simulink model "ProyectoGlobal_AyCD_Cantu_LagoTejo"  (R2021a)
settings: Solver=ode23  StartTime=0.0  StopTime=inf  MinStep=1e-4
values from neighbouring files (symbols this model uses):
  a_hMax = 0.75    [Datos_ProyectoGlobal_AyCD_Cantu_LagoTejo.m]    (also in Datos_v18.m; PID_calculado.mat)
  a_tMax = 0.8    [Datos_ProyectoGlobal_AyCD_Cantu_LagoTejo.m]    (also in Datos_v18.m; PID_calculado.mat)
  b_cx = 1e6    (= 1000000)    [Datos_ProyectoGlobal_AyCD_Cantu_LagoTejo.m]    (also in Datos_v18.m; PID_calculado.mat)
  b_cy = 1e7    (= 10000000)    [Datos_ProyectoGlobal_AyCD_Cantu_LagoTejo.m]    (also in Datos_v18.m; PID_calculado.mat)
  b_eq_h = ((b_hd + b_hm*(i_h^2))*2/(r_hd^2))    (= 31004.4444444)    [Datos_ProyectoGlobal_AyCD_Cantu_LagoTejo.m]    (also in Datos_v18.m; PID_calculado.mat)
  b_eq_t = ((b_td + b_tm*(i_t^2))/(r_td^2))    (= 21607.2)    [Datos_ProyectoGlobal_AyCD_Cantu_LagoTejo.m]    (also in Datos_v18.m; PID_calculado.mat)
  b_hb = 1e8    (= 100000000)    [Datos_ProyectoGlobal_AyCD_Cantu_LagoTejo.m]    (also in Datos_v18.m; PID_calculado.mat)
  b_hEb = 2.2e9    (= 2200000000)    [Datos_ProyectoGlobal_AyCD_Cantu_LagoTejo.m]    (also in Datos_v18.m; PID_calculado.mat)
  b_t = 90    [Datos_ProyectoGlobal_AyCD_Cantu_LagoTejo.m]    (also in Datos_v18.m; PID_calculado.mat)
  b_tb = 5e6    (= 5000000)    [Datos_ProyectoGlobal_AyCD_Cantu_LagoTejo.m]    (also in Datos_v18.m; PID_calculado.mat)
  b_tw = 3e3    (= 3000)    [Datos_ProyectoGlobal_AyCD_Cantu_LagoTejo.m]    (also in Datos_v18.m; PID_calculado.mat)
  b_wu = 150    [Datos_ProyectoGlobal_AyCD_Cantu_LagoTejo.m]    (also in Datos_v18.m; PID_calculado.mat)
  bah = M_eq_h*n_h*omega_h    [PID_Izaje_B.m]    (also in PID_calculado.mat = 387555.555556)
  bat = M_eq_t*n_t*omega_t    [PID_Carro_B.m]    (also in PID_calculado.mat = 270090)
  CI_h = 5    [Datos_ProyectoGlobal_AyCD_Cantu_LagoTejo.m]    (also in Datos_v18.m; PID_calculado.mat)
  CI_t = -16.25    [Datos_ProyectoGlobal_AyCD_Cantu_LagoTejo.m]    (also in Datos_v18.m; PID_calculado.mat)
  d_t = 1e-3    (= 0.001)    [Datos_ProyectoGlobal_AyCD_Cantu_LagoTejo.m]    (also in Datos_v18.m; PID_calculado.mat)
  g = 9.80665    [Datos_ProyectoGlobal_AyCD_Cantu_LagoTejo.m]    (also in Datos_v18.m; PID_calculado.mat)
  H_c = 2.5    [Datos_ProyectoGlobal_AyCD_Cantu_LagoTejo.m]    (also in Datos_v18.m; PID_calculado.mat)
  i_h = 22    [Datos_ProyectoGlobal_AyCD_Cantu_LagoTejo.m]    (also in Datos_v18.m; PID_calculado.mat)
  i_t = 30    [Datos_ProyectoGlobal_AyCD_Cantu_LagoTejo.m]    (also in Datos_v18.m; PID_calculado.mat)
  k_cy = 1.8e9    (= 1800000000)    [Datos_ProyectoGlobal_AyCD_Cantu_LagoTejo.m]    (also in Datos_v18.m; PID_calculado.mat)
  k_tw = 4.8e5    (= 480000)    [Datos_ProyectoGlobal_AyCD_Cantu_LagoTejo.m]    (also in Datos_v18.m; PID_calculado.mat)
  k_wu = 2.36e8    (= 236000000)    [Datos_ProyectoGlobal_AyCD_Cantu_LagoTejo.m]    (also in Datos_v18.m; PID_calculado.mat)
  Kd_bal = [-2.22044604925e-16 2.22044604925e-16 2.22044604925e-16 0 0 0 0 0 -2.22044604925e-16 0 2.22044604925e-16 -2.22044604925e-16 ... (296091 elements, 501x591)]    [Kp_Kd_balanceo.mat]    (also in PD_Balanceo.m = zeros(length(ML),length(L)))
  Kp_bal = [5.11381136401 5.1081388039 5.10248507909 5.09685008556 5.09123372013 5.08563588037 5.08005646467 5.07449537218 5.06895250283 5.06342775732 5.05792103709 5.05243224433 ... (296091 elements, 501x591)]    [Kp_Kd_balanceo.mat]    (also in PD_Balanceo.m = Kd_bal)
  ksah = M_eq_h*n_h*(omega_h^2)    [PID_Izaje_B.m]    (also in PID_calculado.mat = 922348.374575)
  ksat = M_eq_t*n_t*(omega_t^2)    [PID_Carro_B.m]    (also in PID_calculado.mat = 972648.108)
  ksiah = M_eq_h*n_h*(omega_h^3)    [PID_Izaje_B.m]    (also in PID_calculado.mat = 2195108.57705)
  ksiat = M_eq_t*n_t*(omega_t^3)    [PID_Carro_B.m]    (also in PID_calculado.mat = 3502700.36653)
  lim_xDer = 50    [Datos_ProyectoGlobal_AyCD_Cantu_LagoTejo.m]    (also in Datos_v18.m; PID_calculado.mat)
  lim_xDer_ult = 51    [Datos_ProyectoGlobal_AyCD_Cantu_LagoTejo.m]    (also in Datos_v18.m; PID_calculado.mat)
  lim_xIzq = -30    [Datos_ProyectoGlobal_AyCD_Cantu_LagoTejo.m]    (also in Datos_v18.m; PID_calculado.mat)
  lim_xIzq_ult = -31    [Datos_ProyectoGlobal_AyCD_Cantu_LagoTejo.m]    (also in Datos_v18.m; PID_calculado.mat)
  lim_yInf = -20    [Datos_ProyectoGlobal_AyCD_Cantu_LagoTejo.m]    (also in Datos_v18.m; PID_calculado.mat)
  lim_yInf_ult = -21    [Datos_ProyectoGlobal_AyCD_Cantu_LagoTejo.m]    (also in Datos_v18.m; PID_calculado.mat)
  lim_ySup = 40    [Datos_ProyectoGlobal_AyCD_Cantu_LagoTejo.m]    (also in Datos_v18.m; PID_calculado.mat)
  lim_ySup_ult = 41    [Datos_ProyectoGlobal_AyCD_Cantu_LagoTejo.m]    (also in Datos_v18.m; PID_calculado.mat)
  M_cMax = 50000    [Datos_ProyectoGlobal_AyCD_Cantu_LagoTejo.m]    (also in Datos_v18.m; PID_calculado.mat)
  M_cMin = 2000    [Datos_ProyectoGlobal_AyCD_Cantu_LagoTejo.m]    (also in Datos_v18.m; PID_calculado.mat)
  M_eq_h = (J_hd_hEb+J_hm_hb*i_h^2)*2/r_hd^2    (= 65137.7777778)    [Datos_ProyectoGlobal_AyCD_Cantu_LagoTejo.m]    (also in Datos_v18.m; PID_calculado.mat)
  M_l_max = 32500    [Datos_ProyectoGlobal_AyCD_Cantu_LagoTejo.m]    (also in Datos_v18.m; PID_calculado.mat)
  M_l_nom = 65000    [Datos_ProyectoGlobal_AyCD_Cantu_LagoTejo.m]    (also in Datos_v18.m; PID_calculado.mat)
  M_s = 15000    [Datos_ProyectoGlobal_AyCD_Cantu_LagoTejo.m]    (also in Datos_v18.m; PID_calculado.mat)
  M_t = 30000    [Datos_ProyectoGlobal_AyCD_Cantu_LagoTejo.m]    (also in Datos_v18.m; PID_calculado.mat)
  P_h_nom = 956.15e3    (= 956150)    [Datos_ProyectoGlobal_AyCD_Cantu_LagoTejo.m]    (also in Datos_v18.m; PID_calculado.mat)
  r_hd = 0.75    [Datos_ProyectoGlobal_AyCD_Cantu_LagoTejo.m]    (also in Datos_v18.m; PID_calculado.mat)
  r_td = 0.5    [Datos_ProyectoGlobal_AyCD_Cantu_LagoTejo.m]    (also in Datos_v18.m; PID_calculado.mat)
  T_hbMax = 5e4    (= 50000)    [Datos_ProyectoGlobal_AyCD_Cantu_LagoTejo.m]    (also in Datos_v18.m; PID_calculado.mat)
  T_hEbMax = 1.1e6    (= 1100000)    [Datos_ProyectoGlobal_AyCD_Cantu_LagoTejo.m]    (also in Datos_v18.m; PID_calculado.mat)
  T_hmMax = 2e4    (= 20000)    [Datos_ProyectoGlobal_AyCD_Cantu_LagoTejo.m]    (also in Datos_v18.m; PID_calculado.mat)
  T_tbMax = 5e3    (= 5000)    [Datos_ProyectoGlobal_AyCD_Cantu_LagoTejo.m]    (also in Datos_v18.m; PID_calculado.mat)
  T_tmMax = 3e3    (= 3000)    [Datos_ProyectoGlobal_AyCD_Cantu_LagoTejo.m]    (also in Datos_v18.m; PID_calculado.mat)
  tau_hm = 1e-3    (= 0.001)    [Datos_ProyectoGlobal_AyCD_Cantu_LagoTejo.m]    (also in Datos_v18.m; PID_calculado.mat)
  tau_tm = 1e-3    (= 0.001)    [Datos_ProyectoGlobal_AyCD_Cantu_LagoTejo.m]    (also in Datos_v18.m; PID_calculado.mat)
  v_hMax_0 = 3    [Datos_ProyectoGlobal_AyCD_Cantu_LagoTejo.m]    (also in Datos_v18.m; PID_calculado.mat)
  v_hMax_l = 1.5    [Datos_ProyectoGlobal_AyCD_Cantu_LagoTejo.m]    (also in Datos_v18.m; PID_calculado.mat)
  v_tMax = 4    [Datos_ProyectoGlobal_AyCD_Cantu_LagoTejo.m]    (also in Datos_v18.m; PID_calculado.mat)
  xc = [-28.75 -26.25 -23.75 -21.25 -18.75 -16.25 -13.75 -11.25 -8.75 -6.25 -3.75 -1.25 ... (32 elements, 1x32)]    [PID_calculado.mat]    (also in Perfil_Carga.m = -30+1.25:2.5:50-1.25)
  Y_sb = 15    [Datos_ProyectoGlobal_AyCD_Cantu_LagoTejo.m]    (also in Datos_v18.m; PID_calculado.mat)
  Y_t0 = 45    [Datos_ProyectoGlobal_AyCD_Cantu_LagoTejo.m]    (also in Datos_v18.m; PID_calculado.mat)
  yc = [0 0 0 2.5 0 2.5 0 2.5 0 0 0 0 ... (32 elements, 1x32)]    [PID_calculado.mat]    (also in Perfil_Carga.m = yc2)
undefined symbols (not defined in the file or in its folder): b_eq_td, M_eq_td
libraries: simulink x13
(part 1 of 2)
settings Model: SimulationMode=accelerator  PacingRate=5  Creator=Maxi  LastModifiedBy=maxim
settings SolverCC: InitialStep=1e-3  MaxConsecutiveZCs=10000  MaxConsecutiveMinStep=10000000  ZeroCrossAlgorithm=Adaptive  AlgebraicLoopSolver=TrustRegion
settings DebuggingCC: AlgebraicLoopMsg=none  MaskedZcDiagnostic=none  IgnoredZcDiagnostic=none  SFUnusedDataAndEventsDiag=none  UnderSpecifiedDimensionMsg=warning
settings RTWCC: DLArmComputeVersion=20.02.1

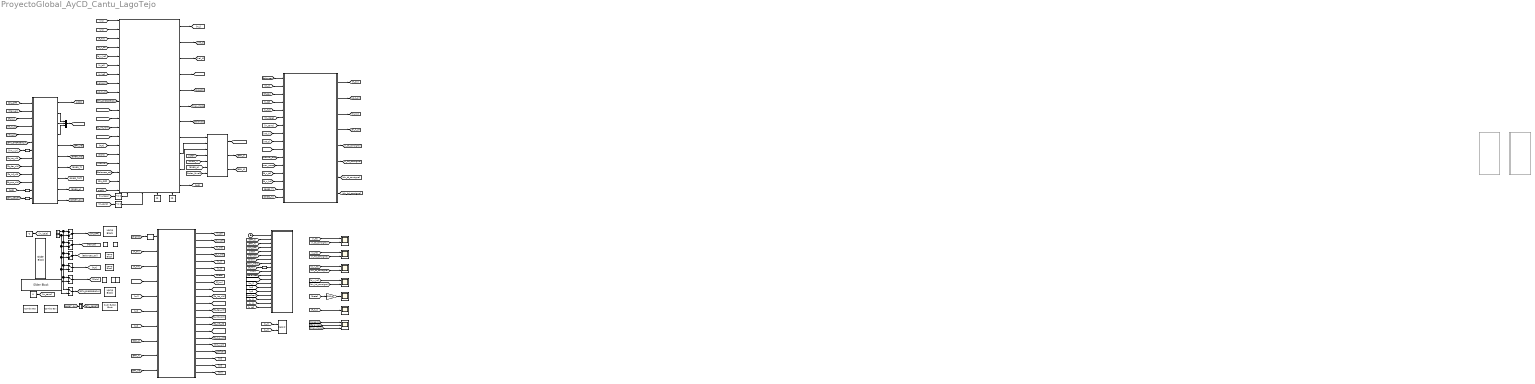
== system ProyectoGlobal_AyCD_Cantu_LagoTejo ==
  note: VISUALIZACION
  note: NIVEL 2
  note: SISTEMA FÍSICO
  note: NIVEL 1
  note: NIVEL 0
  note: HMI
  "  Do" : LampBlock  LabelPosition=Hide
  Angulo de balanceo : Scope
  Automático : LampBlock  LabelPosition=Hide
  Balanceo : LampBlock  LabelPosition=Hide
  Carril Fin : ComboBox  LabelPosition=Hide  SelectedLabel=16
      settings: Values={{'1', '2', '3', '4', '5', '6', '7', '8', '9', '10', '11', '12', '13', '14', '15', '16', '17', '18'}, [1 2 3 4 5 6 7 8 9 10 11 12 13 14 15 16 17 18]}
  Carril Fin Doble : ComboBox  LabelPosition=Hide  SelectedLabel=16
      settings: Values={{'1', '2', '3', '4', '5', '6', '7', '8', '9', '10', '11', '12', '13', '14', '15', '16', '17', '18'}, [1 2 3 4 5 6 7 8 9 10 11 12 13 14 15 16 17 18]}
  Clock2 : Clock
  Compare To Zero : simulink/Logic and Bit Operations/Compare To Zero  relop=>  OutDataTypeStr=boolean
  Compare To Zero2 : simulink/Logic and Bit Operations/Compare To Zero  relop=~=  OutDataTypeStr=boolean
  Compare To Zero7 : simulink/Logic and Bit Operations/Compare To Zero  relop=~=  OutDataTypeStr=boolean
  Constant17 : Constant  Value=0
  Constant18 : Constant
  EMERGENCIA : LampBlock  LabelPosition=Hide
  ENCENDIDO : LampBlock  LabelPosition=Hide
  Estado Final de Frenos : Subsystem
  Estado Final de Frenos10 : Subsystem  Commented=on
  Estado Final de Frenos2 : Subsystem  Commented=on
  Fuerza cable de izaje : Scope
  Gain3 : Gain  Gain=180/pi
  Izaje de carga : Scope  NumInputPorts=2
  MATLAB Function1 : MATLAB Function  TreatAsAtomicUnit=on
  Manual : LampBlock  LabelPosition=Hide
  Manual Switch1 : ManualSwitch  CurrentSetting=0
  Manual Switch2 : ManualSwitch  CurrentSetting=0
  Manual Switch3 : ManualSwitch
  Manual Switch4 : ManualSwitch  CurrentSetting=0
  Manual Switch5 : ManualSwitch
  Manual Switch7 : ManualSwitch
  Memory{5,10,12..13} (4 alike) : Memory
  Modelo Fisico Carro-Izaje-Carga : Subsystem
  Mux7 : Mux  Inputs=3
  Nivel 0 : Stateflow chart  TreatAsAtomicUnit=on
      settings: PortSchema="{\"entries\":[{\"content\":{\"sides\":[{\"content\":{\"connectorIds\":[\"In6\",\"In7\",\"In5\",\"In2\",\"In1\",\"In3\",\"In4\",\"In8\",\"In9\",\"In10\",\"In11\",\"In12\",\"In13\"]},\"type\":\"ConnectorPlacement.EquallySpacedRectSide\",\"uuid\":\"e3679c49-321c-4245-9f4d-6b72d70eef8d\"},{\"content\":{\"connectorIds\":[\"Out1\",\"Out3\",\"Out5\",\"Out4\",\"Out2\",\"Out6\",\"Out7\",\"Out8\",\"Out9\",\"Out10\"],\"side\":\"RIGHT\"},\"type\":\"ConnectorPlacement.EquallySpacedRectSide\",\"uuid\":\"16418e5e-e28d-455d-933a-43b8d78ab460\"},{\"content\":{\"connectorIds\":[],\"side\":\"TOP\"},\"type\":\"ConnectorPlacement.EquallySpacedRectSide\",\"uuid\":\"c85d7e80-ad5f-4217-ba10-6288ee566bb8\"}]},\"type\":\"ConnectorPlacement.EquallySpacedConnector\",\"uuid\":\"c38c6e76-5322-4b57-8473-560e5b1141d3\"}],\"packageUris\":[\"http://schema.mathworks.com/mf0/Connector/R2020b\"],\"version\":\"1.0\"}"
  Nivel 1 : Stateflow chart  TreatAsAtomicUnit=on
      settings: PortSchema="{\"entries\":[{\"content\":{\"sides\":[{\"content\":{\"connectorIds\":[\"In22\",\"In21\",\"In11\",\"In20\",\"In19\",\"In9\",\"In10\",\"In8\",\"In4\",\"In13\",\"In15\",\"In16\",\"In17\",\"In18\",\"In3\",\"In14\",\"In12\",\"In5\",\"In6\",\"In7\"]},\"type\":\"ConnectorPlacement.EquallySpacedRectSide\",\"uuid\":\"68c99711-1ca5-49d6-a421-ad202abad7a3\"},{\"content\":{\"connectorIds\":[\"Out5\",\"Out8\",\"Out6\",\"Out7\",\"Out9\",\"Out11\",\"Out2\",\"Out3\",\"Out4\",\"Out1\",\"Out10\"],\"side\":\"RIGHT\"},\"type\":\"ConnectorPlacement.EquallySpacedRectSide\",\"uuid\":\"bc0f262a-18b8-4d7b-9b7f-403e0cd3788b\"},{\"content\":{\"connectorIds\":[],\"side\":\"TOP\"},\"type\":\"ConnectorPlacement.EquallySpacedRectSide\",\"uuid\":\"2d69c358-e680-43cc-a1d0-9fcf2b39de17\"},{\"content\":{\"connectorIds\":[\"In1\",\"In2\",\"In23\",\"In24\"],\"side\":\"BOTTOM\"},\"type\":\"ConnectorPlacement.EquallySpacedRectSide\",\"uuid\":\"d4a5b5d0-6661-40f6-8d98-5cae5bd8c928\"}]},\"type\":\"ConnectorPlacement.EquallySpacedConnector\",\"uuid\":\"d3c5d26b-109c-4d02-96fa-92f2f1f71ce2\"}],\"packageUris\":[\"http://schema.mathworks.com/mf0/Connector/R2020b\"],\"version\":\"1.0\"}"
  Nivel 2 : Subsystem
  Push Button1 : PushButtonBlock  ButtonText=RESET
  Record : Record  FileSettingsInternal="{\"entries\":[{\"content\":{\"excelSettings\":{\"content\":{},\"type\":\"Streamout.ExcelSettings\"}},\"type\":\"Streamout.FileSettingStorage\",\"uuid\":\"bed3a6e0-7c45-46bb-b7f7-e86d5775e973\"}],\"packageUris\":[\"http://schema.mathworks.com/mf0/streamout_blocks/R2020a\"],\"version\":\"1.0\"}"  Layout=[1 1]  SignalsInternal="{\"entries\":[{\"content\":{\"signals\":[{\"content\":{\"blockPath\":[\"ProyectoGlobal_AyCD_Cantu_LagoTejo/Record\"],\"channel\":[],\"dimensions\":[1],\"domain\":\"proyectoglobal_aycd_cantu_lagotejo/record\",\"lineColor\":\"#ff6929\",\"plots\":[1],\"port\":1,\"sid\":[],\"signalID\":9,\"signalName\":\"x_l\"},\"type\":\"RecordBlkView.Signal\",\"uuid\":\"2278e07a-91c8-4deb-bc74-502acb9eaad0\"},{\"content\":{\"blockPath\":[\"ProyectoGlobal_AyCD_Cantu_LagoTejo/Record\"],\"channel\":[],\"dimensions\":[1],\"domain\":\"proyectoglobal_aycd_cantu_lagotejo/record\",\"lineColor\":\"#b746ff\",\"plots\":[1],\"port\":2,\"sid\":[],\"signalID\":12,\"signalName\":\"y_l\"},\"type\":\"RecordBlkView.Signal\",\"uuid\":\"c595ba9b-7864-403c-ab0d-c6443858467c\"}]},\"type\":\"RecordBlkView.InputSignals\",\"uuid\":\"579f4fff-b8b9-4a59-ac91-7ba26af83972\"}],\"packageUris\":[\"http://schema.mathworks.com/mf0/streamout_blocks/R2020a\"],\"version\":\"1.0\"}"  VisualizationBindings="{\"xyplotplugin\":{\"info\":[{\"series\":[{\"bindingParametersList\":[{\"parameter\":\"Y-Axis\",\"signalID\":12,\"signalName\":\"y_l\"},{\"parameter\":\"X-Axis\",\"signalID\":9,\"signalName\":\"x_l\"}],\"seriesID\":935}],\"subplotID\":1}]}}"
  Scope1 : Scope  NumInputPorts=3
  Simple : LampBlock  LabelPosition=Hide
  Slider : SliderBlock  ScaleMin=-3  ScaleMax=3  TickInterval=1
  Slider1 : SliderBlock  ScaleMin=-4  ScaleMax=+4  TickInterval=1
  Subsystem : Subsystem
  Traslacion de carga : Scope  NumInputPorts=2
  Twistlocks : LampBlock  LabelPosition=Hide
  Velocidad de izaje carga : Scope  NumInputPorts=2
  Velocidad de traslacion carga : Scope  NumInputPorts=2
  "ble   " : LampBlock  LabelPosition=Hide
  carril_fin : Constant  Value=16
  carril_finDoble : Constant  Value=16
  in_carro : Constant  Value=0
  in_izaje : Constant  Value=-2
  tag scope: Orden_Nivel0=global, sistOK=global
  wires:
  Modelo Fisico Carro-Izaje-Carga/1(x_td) -> [x_td]
  Modelo Fisico Carro-Izaje-Carga/3(x_hd) -> [x_hd]
  Modelo Fisico Carro-Izaje-Carga/7(theta) -> [theta]
  [yc] -> Modelo Fisico Carro-Izaje-Carga/6(Yc)
  Modelo Fisico Carro-Izaje-Carga/5(x_l) -> [x_l]
  Modelo Fisico Carro-Izaje-Carga/6(y_l) -> [y_l]
  Modelo Fisico Carro-Izaje-Carga/8(F_hw) -> [F_hw]
  Modelo Fisico Carro-Izaje-Carga/2(d_x_td) -> [d_x_td]
  Modelo Fisico Carro-Izaje-Carga/4(d_x_hd) -> [d_x_hd]
  [T_tm] -> Modelo Fisico Carro-Izaje-Carga/2(T_tm)
  [T_hm] -> Modelo Fisico Carro-Izaje-Carga/3(T_hm)
  [ml] -> Modelo Fisico Carro-Izaje-Carga/5(m_l)
  [theta] -> Gain3/1  "Angulo de balanceo"
  [dx_hd_consigna] -> Velocidad de izaje carga/2  "vel_y_carga*"
  [d_x_td] -> Velocidad de traslacion carga/1  "vel_X_carga"
  [x_hd_consigna] -> Izaje de carga/2  "Y_carga*"
  [d_x_hd] -> Velocidad de izaje carga/1  "vel_Y_carga"
  [x_td] -> Traslacion de carga/1  "X_carga"
  [x_td_consigna] -> Traslacion de carga/2  "X_carga*"
  [x_hd] -> Izaje de carga/1  "Y_carga"
  [dx_td_consigna] -> Velocidad de traslacion carga/2  "vel_X_carga*"
  Gain3/1 -> Angulo de balanceo/1
  [BRK_h] -> Modelo Fisico Carro-Izaje-Carga/9(BRK_h)
  [BRK_hE] -> Modelo Fisico Carro-Izaje-Carga/10(BRK_hE)
  [BRK_t] -> Modelo Fisico Carro-Izaje-Carga/8(BRK_t)
  Modelo Fisico Carro-Izaje-Carga/14(fc_inf_ult) -> [fc_inf_ult]
  Modelo Fisico Carro-Izaje-Carga/17(lim_v_h) -> [lim_v_h]
  [cargado] -> Memory5/1
  Memory5/1 -> Modelo Fisico Carro-Izaje-Carga/1(TLK)
  Modelo Fisico Carro-Izaje-Carga/13(fc_inf_norm) -> [fc_inf_norm]
  Modelo Fisico Carro-Izaje-Carga/16(fc_sup_ult) -> [fc_sup_ult]
  Modelo Fisico Carro-Izaje-Carga/12(fc_der_ult) -> [fc_der_ult]
  Modelo Fisico Carro-Izaje-Carga/9(fc_izq_norm) -> [fc_izq_norm]
  Modelo Fisico Carro-Izaje-Carga/10(fc_izq_ult) -> [fc_izq_ult]
  Modelo Fisico Carro-Izaje-Carga/11(fc_der_norm) -> [fc_der_norm]
  Modelo Fisico Carro-Izaje-Carga/15(fc_sup_norm) -> [fc_sup_norm]
  [xc] -> Modelo Fisico Carro-Izaje-Carga/7(Xc)
  [vel_hMax] -> Modelo Fisico Carro-Izaje-Carga/4(vel_hMax)
  [x_l] -> Record/1
  [y_l] -> Record/2
  [fc_inf_norm] -> Nivel 1/17(fc_inf_norm)
  [vel_t_on] -> Nivel 1/8(vel_t_on)
  [sistOK] -> Nivel 1/7(sistOK)
  Nivel 1/10(WD) -> [WD]
  [fc_der_norm] -> Nivel 1/16(fc_der_norm)
  [ON_OFF] -> Nivel 1/6(ON_OFF)
  Nivel 1/7(vel_hMax) -> [vel_hMax]
  carril_fin/1 -> Nivel 1/23(carril_fin)
  [d_x_hd] -> Nivel 1/19(d_x_h)
  [x_td] -> Nivel 1/9(x_td)
  [F_hw] -> Nivel 1/11(F_hw)
  [fc_izq_norm] -> Nivel 1/15(fc_izq_norm)
  Nivel 1/9(cargado) -> [cargado]
  [TLK] -> Nivel 1/3(TLK)
  [d_x_td] -> Nivel 1/20(d_x_t)
  [Ciclo] -> Nivel 1/14(Ciclo_Doble)
  [Manual] -> Nivel 1/12(Manual)
  [Balanceo_ctrl] -> Nivel 1/5(Balanceo_ctrl)
  Nivel 1/2(Balanceo) -> [Balanceo]
  [x_hd] -> Nivel 1/10(x_hd)
  [xc] -> Nivel 1/22(Xc)
  [yc] -> Nivel 1/21(Yc)
  Nivel 1/5(m_l) -> [m_l]
  [fc_sup_norm] -> Nivel 1/18(fc_sup_norm)
  Nivel 1/6(vel_h) -> [vel_h]
  [vel_h_on] -> Nivel 1/4(vel_h_on)
  Nivel 1/8(vel_t) -> [vel_t]
  carril_finDoble/1 -> Nivel 1/24(carril_finDoble)
  [m_l] -> Nivel 2/2(m_l)
  [x_hd] -> Nivel 2/5(x_hd)
  Nivel 2/5(x_td*) -> [x_td_consigna]
  Nivel 2/2(vel_t_on) -> [vel_t_on]
  Nivel 2/4(vel_h_on) -> [vel_h_on]
  [Balanceo] -> Nivel 2/1(Balanceo_ctrl)
  Nivel 2/6(x_hd*) -> [x_hd_consigna]
  Nivel 2/8(d_x_hd*) -> [dx_hd_consigna]
  Nivel 2/1(T_tm) -> [T_tm]
  Nivel 2/3(T_hm) -> [T_hm]
  [vel_h] -> Nivel 2/8(vel_h)
  [x_td] -> Nivel 2/4(x_td)
  [in_izaje] -> Nivel 2/6(in_izaje)
  Nivel 2/7(d_x_td*) -> [dx_td_consigna]
  [theta] -> Nivel 2/3(theta)
  [vel_hMax] -> Nivel 2/10(vel_hMax)
  [in_carro] -> Nivel 2/7(in_carro)
  [max_masa] -> Nivel 2/12(max_masa)
  [manual_auto] -> Nivel 2/11(manual_auto)
  [vel_t] -> Nivel 2/9(vel_t)
  Compare To Zero7/1 -> Nivel 1/2(in_carro_on)
  [in_carro] -> Compare To Zero7/1
  Compare To Zero2/1 -> Nivel 1/1(in_izaje_on)
  [in_izaje] -> Compare To Zero2/1
  [vel_t_on] -> Nivel 0/1(vel_t_on)
  Nivel 0/10(RESET_OK) -> [RESET_OK]
  [vel_h_on] -> Nivel 0/2(vel_h_on)
  [fc_izq_ult] -> Nivel 0/8(fc_izq_ult)
  Mux7/1 -> [Orden_Nivel0]
  Nivel 0/5(BRK_t) -> Mux7/2
  [Manual] -> Nivel 0/7(MANUAL)
  [ON_OFF] -> Nivel 0/6(ON_OFF)
  Nivel 0/9(EMER_H) -> [EMER_H]
  [lim_v_h] -> Memory12/1
  [BTN_RESET] -> Memory10/1
  [fc_der_ult] -> Nivel 0/9(fc_der_ult)
  Nivel 0/1(sistOK) -> [sistOK]
  Nivel 0/8(EMER_TOT) -> [EMER_TOT]
  Nivel 0/4(BRK_h) -> Mux7/3
  [BTN_EMERGENCIA] -> Nivel 0/3(BTN_EMERGENCIA)
  Memory12/1 -> Nivel 0/4(lim_v_h)
  Memory13/1 -> Nivel 0/12(WD)
  Nivel 0/3(manual_auto) -> Mux7/1
  Nivel 0/7(EMER_T) -> [EMER_T]
  [WD] -> Memory13/1
  Nivel 0/6(EMER_WD) -> [EMER_WD]
  [fc_inf_ult] -> Nivel 0/10(fc_inf_ult)
  Nivel 0/2(BRK_hE) -> [BRK_hE]
  [F_hw] -> Nivel 0/5(F_hw)
  [fc_sup_ult] -> Nivel 0/11(fc_sup_ult)
  Modelo Fisico Carro-Izaje-Carga/18(graficar) -> [graficar]
  Modelo Fisico Carro-Izaje-Carga/19(xc) -> [xc]
  Modelo Fisico Carro-Izaje-Carga/20(yc) -> [yc]
  Modelo Fisico Carro-Izaje-Carga/21(m_l_real) -> [ml]
  Nivel 1/11(max_masa) -> [max_masa]
  Memory10/1 -> Nivel 0/13(BTN_RESET)
  [BTN_EMERGENCIA] -> Nivel 1/13(BTN_EMERGENCIA)
  [F_hw] -> Fuerza cable de izaje/1  "F_hw"
  [cargado] -> Scope1/1  "cargado"
  [Balanceo] -> Scope1/2  "Balanceo"
  [max_masa] -> Scope1/3  "max_masa"
  [d_x_td] -> Nivel 2/13(d_x_td)
  [d_x_hd] -> Nivel 2/14(d_x_hd)
  [BRK_h] -> MATLAB Function1/3(BRK_h)
  [BRK_t] -> MATLAB Function1/2(BRK_t)
  [yc] -> MATLAB Function1/15(yc)
  [max_masa] -> MATLAB Function1/8(max_masa)
  [Balanceo] -> MATLAB Function1/11(Balanceo)
  [x_l] -> MATLAB Function1/17(x_l)
  [xc] -> MATLAB Function1/14(xc)
  [Manual] -> MATLAB Function1/6(Manual)
  [Ciclo] -> MATLAB Function1/7(Ciclo)
  Compare To Zero/1 -> MATLAB Function1/9(Tension_hw)
  [ON_OFF] -> MATLAB Function1/4(ON_OFF)
  [manual_auto] -> MATLAB Function1/12(manual_auto)
  [y_l] -> MATLAB Function1/18(y_l)
  Clock2/1 -> MATLAB Function1/1(clock)
  [x_td] -> MATLAB Function1/19(x_td)
  [TLK] -> MATLAB Function1/10(TLK)
  [sistOK] -> MATLAB Function1/5(sist_OK)
  [m_l] -> MATLAB Function1/13(ml_medida)
  [graficar] -> MATLAB Function1/16(graficar)
  Constant18/1 -> Manual Switch2/2, Manual Switch4/2, Manual Switch3/2, Manual Switch7/2, Manual Switch5/2, Manual Switch1/2
  Manual Switch2/1 -> [Manual]
  Manual Switch5/1 -> [Ciclo]
  [RESET_OK] -> Subsystem/1(" ")
  Manual Switch7/1 -> [BTN_EMERGENCIA]
  Constant17/1 -> Manual Switch2/1, Manual Switch4/1, Manual Switch3/1, Manual Switch7/1, Manual Switch5/1, Manual Switch1/1
  Subsystem/1(Out1) -> [BTN_RESET]
  in_izaje/1 -> [in_izaje]
  in_carro/1 -> [in_carro]
  Manual Switch1/1 -> [ON_OFF]
  Manual Switch4/1 -> [Balanceo_ctrl]
  Manual Switch3/1 -> [TLK]
  [EMER_H] -> Estado Final de Frenos/6(EMER_h)
  Estado Final de Frenos/1(manual_auto_def) -> [manual_auto]
  Estado Final de Frenos/2(BRK_t_def) -> [BRK_t]
  Estado Final de Frenos/3(BRK_h_def) -> [BRK_h]
  [Orden_Nivel0] -> Estado Final de Frenos/7(Orden_Nivel0)
  [EMER_T] -> Estado Final de Frenos/5(EMER_T)
  [sistOK] -> Estado Final de Frenos/4(sistOK)
  Nivel 1/1(BRK_h) -> Estado Final de Frenos/3(BRK_h)
  Nivel 1/4(BRK_t) -> Estado Final de Frenos/2(BRK_t)
  Nivel 1/3(manual_auto) -> Estado Final de Frenos/1(manual_auto_Nivel1)
  [EMER_T] -> Nivel 2/15(EMER_T)
  [EMER_H] -> Nivel 2/16(EMER_H)
  [F_hw] -> Compare To Zero/1

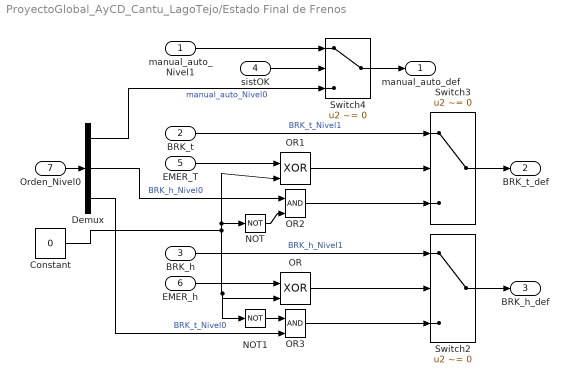
== system ProyectoGlobal_AyCD_Cantu_LagoTejo/Estado Final de Frenos ==
  manual_auto_Nivel1 : Inport
  BRK_t : Inport  Port=2
  BRK_h : Inport  Port=3
  sistOK : Inport  Port=4
  EMER_T : Inport  Port=5
  EMER_h : Inport  Port=6
  Orden_Nivel0 : Inport  Port=7
  Constant : Constant  Value=0
  Demux : Demux  Outputs=3
  NOT : Logic  Operator=NOT  IconShape=distinctive  AllPortsSameDT=off  OutDataTypeStr=boolean
  NOT1 : Logic  Operator=NOT  IconShape=distinctive  AllPortsSameDT=off  OutDataTypeStr=boolean
  OR : Logic  Operator=XOR  IconShape=distinctive  AllPortsSameDT=off  OutDataTypeStr=boolean
  OR1 : Logic  Operator=XOR  IconShape=distinctive  AllPortsSameDT=off  OutDataTypeStr=boolean
  OR2 : Logic  IconShape=distinctive  AllPortsSameDT=off  OutDataTypeStr=boolean
  OR3 : Logic  IconShape=distinctive  AllPortsSameDT=off  OutDataTypeStr=boolean
  Switch2 : Switch  Criteria=u2 ~= 0
  Switch3 : Switch  Criteria=u2 ~= 0
  Switch4 : Switch  Criteria=u2 ~= 0
  manual_auto_def : Outport
  BRK_t_def : Outport  Port=2
  BRK_h_def : Outport  Port=3
  wires:
  NOT1/1 -> OR3/1
  OR3/1 -> Switch2/3
  EMER_h/1 -> OR/1
  NOT/1 -> OR2/2
  OR2/1 -> Switch3/3
  Constant/1 -> NOT/1, OR1/2, OR/2, NOT1/1
  EMER_T/1 -> OR1/1
  Demux/1 -> Switch4/3  "manual_auto_Nivel0"
  Orden_Nivel0/1 -> Demux/1
  Demux/3 -> OR3/2  "BRK_t_Nivel0"
  Demux/2 -> OR2/1  "BRK_h_Nivel0"
  manual_auto_Nivel1/1 -> Switch4/1
  BRK_h/1 -> Switch2/1  "BRK_h_Nivel1"
  BRK_t/1 -> Switch3/1  "BRK_t_Nivel1"
  sistOK/1 -> Switch4/2
  Switch4/1 -> manual_auto_def/1
  Switch2/1 -> BRK_h_def/1
  Switch3/1 -> BRK_t_def/1
  OR1/1 -> Switch3/2
  OR/1 -> Switch2/2

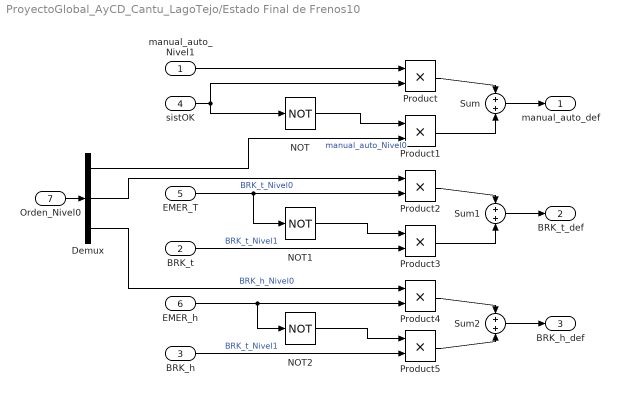
== system ProyectoGlobal_AyCD_Cantu_LagoTejo/Estado Final de Frenos10 ==
  manual_auto_Nivel1 : Inport
  BRK_t : Inport  Port=2
  BRK_h : Inport  Port=3
  sistOK : Inport  Port=4
  EMER_T : Inport  Port=5
  EMER_h : Inport  Port=6
  Orden_Nivel0 : Inport  Port=7
  Demux : Demux  Outputs=3
  NOT : Logic  Operator=NOT  IconShape=distinctive  AllPortsSameDT=off  OutDataTypeStr=boolean
  NOT1 : Logic  Operator=NOT  IconShape=distinctive  AllPortsSameDT=off  OutDataTypeStr=boolean
  NOT2 : Logic  Operator=NOT  IconShape=distinctive  AllPortsSameDT=off  OutDataTypeStr=boolean
  Product{,1..5} (6 alike) : Product
  Sum : Sum  Inputs=+|+
  Sum1 : Sum  Inputs=+|+
  Sum2 : Sum  Inputs=+|+
  manual_auto_def : Outport
  BRK_t_def : Outport  Port=2
  BRK_h_def : Outport  Port=3
  wires:
  Orden_Nivel0/1 -> Demux/1
  Sum/1 -> manual_auto_def/1
  manual_auto_Nivel1/1 -> Product/1
  Product/1 -> Sum/1
  Product1/1 -> Sum/2
  sistOK/1 -> NOT/1, Product/2
  Demux/1 -> Product1/2  "manual_auto_Nivel0"
  NOT/1 -> Product1/1
  Sum1/1 -> BRK_t_def/1
  Product2/1 -> Sum1/1
  Product3/1 -> Sum1/2
  Demux/2 -> Product2/1  "BRK_t_Nivel0"
  EMER_T/1 -> NOT1/1, Product2/2
  NOT1/1 -> Product3/1
  BRK_t/1 -> Product3/2  "BRK_t_Nivel1"
  NOT2/1 -> Product5/1
  Product5/1 -> Sum2/2
  Product4/1 -> Sum2/1
  BRK_h/1 -> Product5/2  "BRK_t_Nivel1"
  Sum2/1 -> BRK_h_def/1
  Demux/3 -> Product4/1  "BRK_h_Nivel0"
  EMER_h/1 -> NOT2/1, Product4/2

== system ProyectoGlobal_AyCD_Cantu_LagoTejo/Estado Final de Frenos2 ==
  manual_auto_Nivel1 : Inport
  BRK_t : Inport  Port=2
  BRK_h : Inport  Port=3
  sistOK : Inport  Port=4
  EMER_T : Inport  Port=5
  EMER_h : Inport  Port=6
  Orden_Nivel0 : Inport  Port=7
  Demux : Demux  Commented=on  Outputs=3
  Switch2 : Switch  Commented=on  Criteria=u2 ~= 0
  Switch3 : Switch  Commented=on  Criteria=u2 ~= 0
  Switch4 : Switch  Commented=on  Criteria=u2 ~= 0
  manual_auto_def : Outport
  BRK_t_def : Outport  Port=2
  BRK_h_def : Outport  Port=3
  wires:
  Demux/3 -> Switch2/1  "BRK_h_Nivel0"
  EMER_T/1 -> Switch3/2
  Demux/2 -> Switch3/1  "BRK_t_Nivel0"
  EMER_h/1 -> Switch2/2
  Demux/1 -> Switch4/3  "manual_auto_Nivel0"
  Orden_Nivel0/1 -> Demux/1
  manual_auto_Nivel1/1 -> Switch4/1
  BRK_h/1 -> Switch2/3  "BRK_h_Nivel1"
  BRK_t/1 -> Switch3/3  "BRK_t_Nivel1"
  sistOK/1 -> Switch4/2
  Switch4/1 -> manual_auto_def/1
  Switch2/1 -> BRK_h_def/1
  Switch3/1 -> BRK_t_def/1

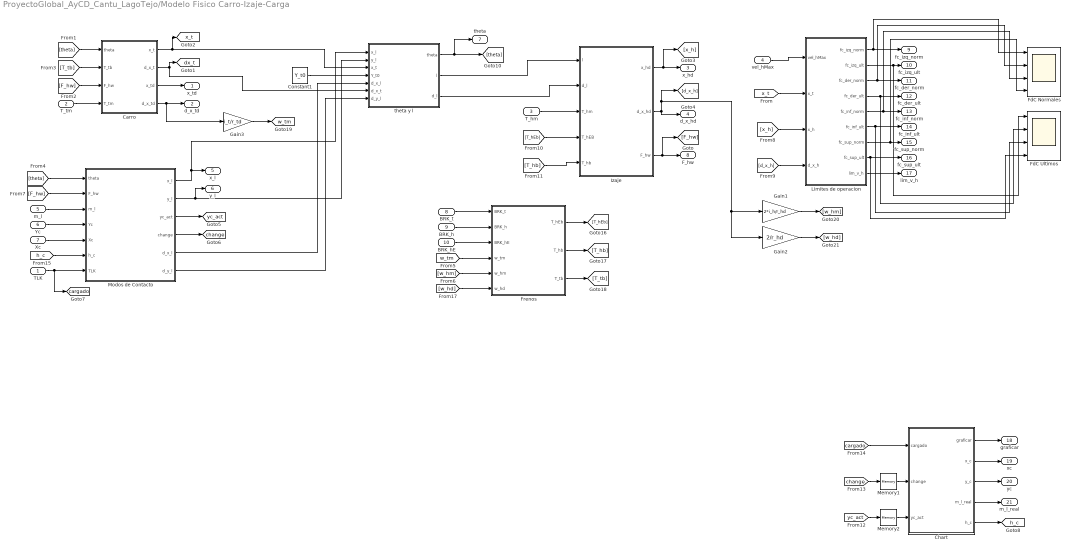
== system ProyectoGlobal_AyCD_Cantu_LagoTejo/Modelo Fisico Carro-Izaje-Carga ==
  TLK : Inport
  T_tm : Inport  Port=2
  T_hm : Inport  Port=3
  vel_hMax : Inport  Port=4
  m_l : Inport  Port=5
  Yc : Inport  Port=6
  Xc : Inport  Port=7
  BRK_t : Inport  Port=8
  BRK_h : Inport  Port=9
  BRK_hE : Inport  Port=10
  Carro : Subsystem
  Chart : Stateflow chart  TreatAsAtomicUnit=on
      settings: PortSchema="{\"entries\":[{\"content\":{\"sides\":[{\"content\":{\"connectorIds\":[\"In1\",\"In2\",\"In3\"]},\"type\":\"ConnectorPlacement.EquallySpacedRectSide\",\"uuid\":\"3e82a7c2-bf75-4f61-8ed8-4dc94ac63b2a\"},{\"content\":{\"connectorIds\":[\"Out3\",\"Out4\",\"Out2\",\"Out5\",\"Out1\"],\"side\":\"RIGHT\"},\"type\":\"ConnectorPlacement.EquallySpacedRectSide\",\"uuid\":\"3bda0d7b-f5b8-4b7e-98a5-641e146bfa09\"},{\"content\":{\"connectorIds\":[],\"side\":\"TOP\"},\"type\":\"ConnectorPlacement.EquallySpacedRectSide\",\"uuid\":\"53c96370-adb7-4c5f-b84b-b565cd95f057\"}]},\"type\":\"ConnectorPlacement.EquallySpacedConnector\",\"uuid\":\"5926f053-77e4-4d2a-97aa-9f275575c8db\"}],\"packageUris\":[\"http://schema.mathworks.com/mf0/Connector/R2020b\"],\"version\":\"1.0\"}"
  Constant1 : Constant  Value=Y_t0
  FdC Normales : Scope  NumInputPorts=4
  FdC Ultimos : Scope  NumInputPorts=4
  Frenos : Subsystem
  Gain1 : Gain  Gain=2*i_h/r_hd
  Gain2 : Gain  Gain=2/r_hd
  Gain3 : Gain  Gain=i_t/r_td
  Izaje : Subsystem
  Limites de operacion : Subsystem
  Memory1 : Memory
  Memory2 : Memory
  Modos de Contacto : Subsystem
  theta y l : Subsystem
  x_td : Outport
  d_x_td : Outport  Port=2
  x_hd : Outport  Port=3
  d_x_hd : Outport  Port=4
  x_l : Outport  Port=5
  y_l : Outport  Port=6
  theta : Outport  Port=7
  F_hw : Outport  Port=8
  fc_izq_norm : Outport  Port=9
  fc_izq_ult : Outport  Port=10
  fc_der_norm : Outport  Port=11
  fc_der_ult : Outport  Port=12
  fc_inf_norm : Outport  Port=13
  fc_inf_ult : Outport  Port=14
  fc_sup_norm : Outport  Port=15
  fc_sup_ult : Outport  Port=16
  lim_v_h : Outport  Port=17
  graficar : Outport  Port=18
  xc : Outport  Port=19
  yc : Outport  Port=20
  m_l_real : Outport  Port=21
  tag scope: cargado=global, change=global, dx_t=global, h_c=global, w_tm=global, x_t=global, yc_act=global
  wires:
  BRK_h/1 -> Frenos/2(BRK_h)
  BRK_t/1 -> Frenos/1(BRK_t)
  BRK_hE/1 -> Frenos/3(BRK_hE)
  [w_tm] -> Frenos/4(w_tm)
  [w_hm] -> Frenos/5(w_hm)
  Limites de operacion/2(fc_izq_ult) -> FdC Ultimos/1, fc_izq_ult/1
  Limites de operacion/1(fc_izq_norm) -> FdC Normales/1, fc_izq_norm/1
  Limites de operacion/6(fc_inf_ult) -> FdC Ultimos/3, fc_inf_ult/1
  Gain2/1 -> [w_hd]
  Limites de operacion/9(lim_v_h) -> lim_v_h/1
  Limites de operacion/3(fc_der_norm) -> FdC Normales/2, fc_der_norm/1
  Limites de operacion/4(fc_der_ult) -> FdC Ultimos/2, fc_der_ult/1
  Limites de operacion/5(fc_inf_norm) -> FdC Normales/3, fc_inf_norm/1
  Gain3/1 -> [w_tm]
  vel_hMax/1 -> Limites de operacion/1(vel_hMax)
  Limites de operacion/8(fc_sup_ult) -> FdC Ultimos/4, fc_sup_ult/1
  Gain1/1 -> [w_hm]
  Frenos/1(T_hEb) -> [T_hEb]
  Frenos/2(T_hb) -> [T_hb]
  Frenos/3(T_tb) -> [T_tb]
  [w_hd] -> Frenos/6(w_hd)
  [theta] -> Carro/1(theta)
  [T_tb] -> Carro/2(T_tb)
  [F_hw] -> Carro/3(F_hw)
  T_tm/1 -> Carro/4(T_tm)
  Carro/2(d_x_t) -> theta y l/6(d_x_t), [dx_t]
  Carro/3(x_td) -> x_td/1
  Carro/4(d_x_td) -> d_x_td/1, Gain3/1
  Modos de Contacto/1(x_l) -> theta y l/1(x_l), x_l/1
  Carro/1(x_t) -> [x_t], theta y l/3(x_t)
  Modos de Contacto/2(y_l) -> y_l/1, theta y l/2(y_l)
  theta y l/1(theta) -> [theta], theta/1
  Constant1/1 -> theta y l/4(Y_t0)
  Modos de Contacto/5(d_x_l) -> theta y l/5(d_x_l)
  Modos de Contacto/6(d_y_l) -> theta y l/7(d_y_l)
  [theta] -> Modos de Contacto/1(theta)
  [F_hw] -> Modos de Contacto/2(F_hw)
  m_l/1 -> Modos de Contacto/3(m_l)
  [h_c] -> Modos de Contacto/6(h_c)
  Yc/1 -> Modos de Contacto/4(Yc)
  Xc/1 -> Modos de Contacto/5(Xc)
  Modos de Contacto/4(change) -> [change]
  [T_hEb] -> Izaje/4(T_hEB)
  T_hm/1 -> Izaje/3(T_hm)
  [T_hb] -> Izaje/5(T_hb)
  theta y l/2(l) -> Izaje/1(l)
  theta y l/3(d_l) -> Izaje/2(d_l)
  Izaje/3(F_hw) -> [F_hw], F_hw/1
  Izaje/1(x_hd) -> [x_h], x_hd/1
  Izaje/2(d_x_hd) -> Gain2/1, Gain1/1, [d_x_h], d_x_hd/1
  [x_t] -> Limites de operacion/2(x_t)
  [x_h] -> Limites de operacion/3(x_h)
  [d_x_h] -> Limites de operacion/4(d_x_h)
  [change] -> Memory1/1
  Chart/1(h_c) -> [h_c]
  Chart/4(x_c) -> xc/1
  Chart/3(graficar) -> graficar/1
  Chart/2(y_c) -> yc/1
  [yc_act] -> Memory2/1
  Modos de Contacto/3(yc_act) -> [yc_act]
  TLK/1 -> [cargado], Modos de Contacto/7(TLK)
  [cargado] -> Chart/1(cargado)
  Memory1/1 -> Chart/2(change)
  Memory2/1 -> Chart/3(yc_act)
  Chart/5(m_l_real) -> m_l_real/1
  Limites de operacion/7(fc_sup_norm) -> FdC Normales/4, fc_sup_norm/1

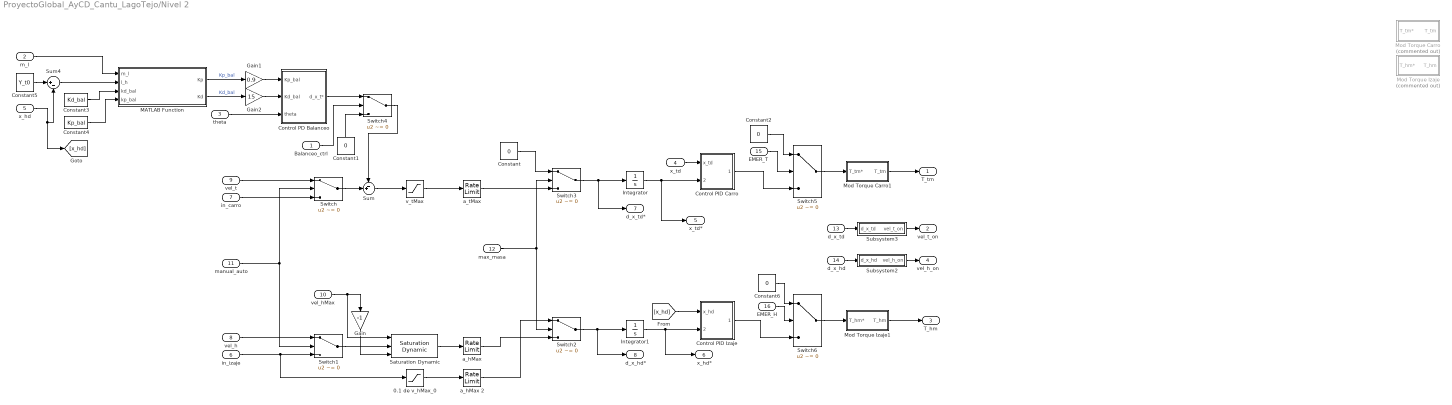
== system ProyectoGlobal_AyCD_Cantu_LagoTejo/Nivel 2 ==
  Balanceo_ctrl : Inport
  m_l : Inport  Port=2
  theta : Inport  Port=3
  x_td : Inport  Port=4
  x_hd : Inport  Port=5
  in_izaje : Inport  Port=6
  in_carro : Inport  Port=7
  vel_h : Inport  Port=8
  vel_t : Inport  Port=9
  vel_hMax : Inport  Port=10
  manual_auto : Inport  Port=11
  max_masa : Inport  Port=12
  d_x_td : Inport  Port=13
  d_x_hd : Inport  Port=14
  EMER_T : Inport  Port=15
  EMER_H : Inport  Port=16
  0.1 de v_hMax_0 : Saturate  UpperLimit=0  LowerLimit=-0.1*v_hMax_0
  Constant{,1..2,6} (4 alike) : Constant  Value=0
  Constant3 : Constant  Value=Kd_bal
  Constant4 : Constant  Value=Kp_bal
  Constant5 : Constant  Value=Y_t0
  Control PD Balanceo : Subsystem
  Control PID Carro : Subsystem
  Control PID Izaje : Subsystem
  Gain : Gain  Gain=-1
  Gain1 : Gain  Gain=0.9
  Gain2 : Gain  Gain=15
  Integrator : Integrator  InitialCondition=CI_t
  Integrator1 : Integrator  InitialCondition=CI_h
  MATLAB Function : MATLAB Function  TreatAsAtomicUnit=on
  Mod Torque Carro : Subsystem  Commented=on
  Mod Torque Carro1 : Subsystem
  Mod Torque Izaje : Subsystem  Commented=on
  Mod Torque Izaje1 : Subsystem
  Saturation Dynamic : simulink/Discontinuities/Saturation Dynamic  OutMin=[]  OutMax=[]  OutDataTypeStr=Inherit: Same as second input  OutDataType=fixdt(1, 16)  OutScaling=2^-10  DoSatur=off
  Subsystem2 : Subsystem
  Subsystem3 : Subsystem
  Sum : Sum  Inputs=-+|
  Sum4 : Sum  Inputs=|+-
  Switch{,1..6} (7 alike) : Switch  Criteria=u2 ~= 0
  a_hMax : RateLimiter  RisingSlewLimit=a_hMax  FallingSlewLimit=-a_hMax  SampleTimeMode=inherited
  a_hMax 2 : RateLimiter  RisingSlewLimit=a_hMax  FallingSlewLimit=-a_hMax  SampleTimeMode=inherited
  a_tMax : RateLimiter  RisingSlewLimit=a_tMax  FallingSlewLimit=-a_tMax  SampleTimeMode=inherited
  v_tMax : Saturate  UpperLimit=v_tMax  LowerLimit=-v_tMax
  T_tm : Outport
  vel_t_on : Outport  Port=2
  T_hm : Outport  Port=3
  vel_h_on : Outport  Port=4
  x_td* : Outport  Port=5
  x_hd* : Outport  Port=6
  d_x_td* : Outport  Port=7
  d_x_hd* : Outport  Port=8
  wires:
  manual_auto/1 -> Switch/2, Switch1/2
  Switch1/1 -> Saturation Dynamic/2
  vel_hMax/1 -> Gain/1, Saturation Dynamic/1
  Gain/1 -> Saturation Dynamic/3
  in_carro/1 -> Switch/3
  vel_h/1 -> Switch1/1
  Saturation Dynamic/1 -> a_hMax/1
  v_tMax/1 -> a_tMax/1
  Constant/1 -> Switch3/1
  0.1 de v_hMax_0/1 -> a_hMax 2/1
  vel_t/1 -> Switch/1
  Switch/1 -> Sum/2
  in_izaje/1 -> 0.1 de v_hMax_0/1, Switch1/3
  max_masa/1 -> Switch3/2, Switch2/2
  a_hMax 2/1 -> Switch2/1
  Sum/1 -> v_tMax/1
  Constant3/1 -> MATLAB Function/3(kd_bal)
  Balanceo_ctrl/1 -> Switch4/2
  Constant4/1 -> MATLAB Function/4(kp_bal)
  Constant5/1 -> Sum4/1
  x_hd/1 -> [x_hd], Sum4/2
  Sum4/1 -> MATLAB Function/2(l_h)
  m_l/1 -> MATLAB Function/1(m_l)
  Constant1/1 -> Switch4/3
  MATLAB Function/1(Kp) -> Gain1/1  "Kp_bal"
  MATLAB Function/2(Kd) -> Gain2/1  "Kd_bal"
  theta/1 -> Control PD Balanceo/3(theta)
  Control PD Balanceo/1(d_x_t*) -> Switch4/1
  x_td/1 -> Control PID Carro/1(x_td)
  Switch2/1 -> d_x_hd*/1, Integrator1/1
  Switch3/1 -> d_x_td*/1, Integrator/1
  Mod Torque Carro1/1(T_tm) -> T_tm/1
  Subsystem3/1(vel_t_on) -> vel_t_on/1
  Integrator/1 -> x_td*/1, Control PID Carro/2(x_td*)
  Integrator1/1 -> Control PID Izaje/2(x_hd*), x_hd*/1
  Mod Torque Izaje1/1(T_hm) -> T_hm/1
  Subsystem2/1(vel_h_on) -> vel_h_on/1
  [x_hd] -> Control PID Izaje/1(x_hd)
  d_x_td/1 -> Subsystem3/1(d_x_td)
  d_x_hd/1 -> Subsystem2/1(d_x_hd)
  Gain1/1 -> Control PD Balanceo/1(Kp_bal)
  Gain2/1 -> Control PD Balanceo/2(Kd_bal)
  Switch4/1 -> Sum/1
  Constant2/1 -> Switch5/1
  Constant6/1 -> Switch6/1
  EMER_T/1 -> Switch5/2
  EMER_H/1 -> Switch6/2
  Control PID Carro/1(T_tm*) -> Switch5/3
  Switch5/1 -> Mod Torque Carro1/1(T_tm*)
  a_tMax/1 -> Switch3/3
  Control PID Izaje/1(T_hm*) -> Switch6/3
  Switch6/1 -> Mod Torque Izaje1/1(T_hm*)
  a_hMax/1 -> Switch2/3

== system ProyectoGlobal_AyCD_Cantu_LagoTejo/Subsystem ==
  " " : Inport
  AND : Logic  IconShape=distinctive  AllPortsSameDT=off  OutDataTypeStr=boolean
  BTN_RESET_PRESSED : Constant  Value=0
  Out1 : Outport
  wires:
  BTN_RESET_PRESSED/1 -> AND/2
  " "/1 -> AND/1
  AND/1 -> Out1/1

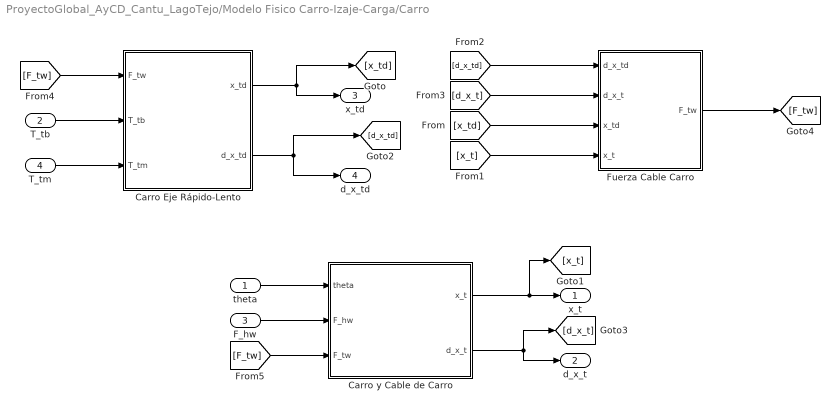
== system ProyectoGlobal_AyCD_Cantu_LagoTejo/Modelo Fisico Carro-Izaje-Carga/Carro ==
  theta : Inport
  T_tb : Inport  Port=2
  F_hw : Inport  Port=3
  T_tm : Inport  Port=4
  Carro Eje Rápido-Lento : Subsystem
  Carro y Cable de Carro : Subsystem
  Fuerza Cable Carro : Subsystem
  x_t : Outport
  d_x_t : Outport  Port=2
  x_td : Outport  Port=3
  d_x_td : Outport  Port=4
  wires:
  T_tb/1 -> Carro Eje Rápido-Lento/2(T_tb)
  theta/1 -> Carro y Cable de Carro/1(theta)
  Carro Eje Rápido-Lento/1(x_td) -> x_td/1, [x_td]
  Carro y Cable de Carro/2(d_x_t) -> [d_x_t], d_x_t/1
  Carro Eje Rápido-Lento/2(d_x_td) -> [d_x_td], d_x_td/1
  F_hw/1 -> Carro y Cable de Carro/2(F_hw)
  Carro y Cable de Carro/1(x_t) -> [x_t], x_t/1
  T_tm/1 -> Carro Eje Rápido-Lento/3(T_tm)
  [x_td] -> Fuerza Cable Carro/3(x_td)
  [x_t] -> Fuerza Cable Carro/4(x_t)
  Fuerza Cable Carro/1(F_tw) -> [F_tw]
  [d_x_td] -> Fuerza Cable Carro/1(d_x_td)
  [d_x_t] -> Fuerza Cable Carro/2(d_x_t)
  [F_tw] -> Carro Eje Rápido-Lento/1(F_tw)
  [F_tw] -> Carro y Cable de Carro/3(F_tw)

== system ProyectoGlobal_AyCD_Cantu_LagoTejo/Modelo Fisico Carro-Izaje-Carga/Frenos ==
  BRK_t : Inport
  BRK_h : Inport  Port=2
  BRK_hE : Inport  Port=3
  w_tm : Inport  Port=4
  w_hm : Inport  Port=5
  w_hd : Inport  Port=6
  Constant : Constant
  Constant1 : Constant  Value=0
  Freno Carro : Subsystem
  Freno Emergencia Izaje : Subsystem
  Freno Izaje : Subsystem
  Manual Switch1 : ManualSwitch
  T_hEb : Outport
  T_hb : Outport  Port=2
  T_tb : Outport  Port=3
  wires:
  Freno Izaje/1(T_hb) -> T_hb/1
  Freno Carro/1(T_tb) -> T_tb/1
  Freno Emergencia Izaje/1(T_hEb) -> T_hEb/1
  w_tm/1 -> Freno Carro/2(w_tm)
  w_hm/1 -> Freno Izaje/2(w_hm)
  w_hd/1 -> Freno Emergencia Izaje/2(w_hd)
  Manual Switch1/1 -> Freno Emergencia Izaje/1(On_Off), Freno Izaje/1(On_Off), Freno Carro/1(On_Off)
  Constant/1 -> Manual Switch1/1
  Constant1/1 -> Manual Switch1/2

== system ProyectoGlobal_AyCD_Cantu_LagoTejo/Modelo Fisico Carro-Izaje-Carga/Izaje ==
  l : Inport
  d_l : Inport  Port=2
  T_hm : Inport  Port=3
  T_hEB : Inport  Port=4
  T_hb : Inport  Port=5
  Fuerza cable de Izaje : Subsystem
  Izaje Eje Rapido-Lento : Subsystem
  x_hd : Outport
  d_x_hd : Outport  Port=2
  F_hw : Outport  Port=3
  wires:
  T_hb/1 -> Izaje Eje Rapido-Lento/4(T_hb)
  T_hEB/1 -> Izaje Eje Rapido-Lento/3(T_hEb)
  [F_hw] -> Izaje Eje Rapido-Lento/1(F_hw)
  T_hm/1 -> Izaje Eje Rapido-Lento/2(T_hm)
  Fuerza cable de Izaje/1(F_hw) -> F_hw/1, [F_hw]
  d_l/1 -> Fuerza cable de Izaje/3(d_l)
  Izaje Eje Rapido-Lento/1(l_h) -> [l_h]
  Izaje Eje Rapido-Lento/3(x_hd) -> x_hd/1
  l/1 -> Fuerza cable de Izaje/1(l)
  Izaje Eje Rapido-Lento/4(d_x_hd) -> d_x_hd/1
  [l_h] -> Fuerza cable de Izaje/2(l_h)
  Izaje Eje Rapido-Lento/2(d_l_h) -> [d_l_h]
  [d_l_h] -> Fuerza cable de Izaje/4(d_l_h)

== system ProyectoGlobal_AyCD_Cantu_LagoTejo/Modelo Fisico Carro-Izaje-Carga/Limites de operacion ==
  vel_hMax : Inport
  x_t : Inport  Port=2
  x_h : Inport  Port=3
  d_x_h : Inport  Port=4
  Límites de Carro : Subsystem
  Subsystem1 : Subsystem
  fc_izq_norm : Outport
  fc_izq_ult : Outport  Port=2
  fc_der_norm : Outport  Port=3
  fc_der_ult : Outport  Port=4
  fc_inf_norm : Outport  Port=5
  fc_inf_ult : Outport  Port=6
  fc_sup_norm : Outport  Port=7
  fc_sup_ult : Outport  Port=8
  lim_v_h : Outport  Port=9
  wires:
  x_t/1 -> Límites de Carro/1(x_t)
  Límites de Carro/1(fc_izq_norm) -> fc_izq_norm/1
  Límites de Carro/2(fc_izq_ult) -> fc_izq_ult/1
  Límites de Carro/3(fc_der_norm) -> fc_der_norm/1
  Límites de Carro/4(fc_der_ult) -> fc_der_ult/1
  Subsystem1/4(fc_sup_ult) -> fc_sup_ult/1
  Subsystem1/3(fc_sup_norm) -> fc_sup_norm/1
  Subsystem1/2(fc_inf_ult) -> fc_inf_ult/1
  Subsystem1/1(fc_inf_norm) -> fc_inf_norm/1
  x_h/1 -> Subsystem1/1(x_h)
  d_x_h/1 -> Subsystem1/3(d_x_h)
  Subsystem1/5(lim_v_h) -> lim_v_h/1
  vel_hMax/1 -> Subsystem1/2(vel_hMax)

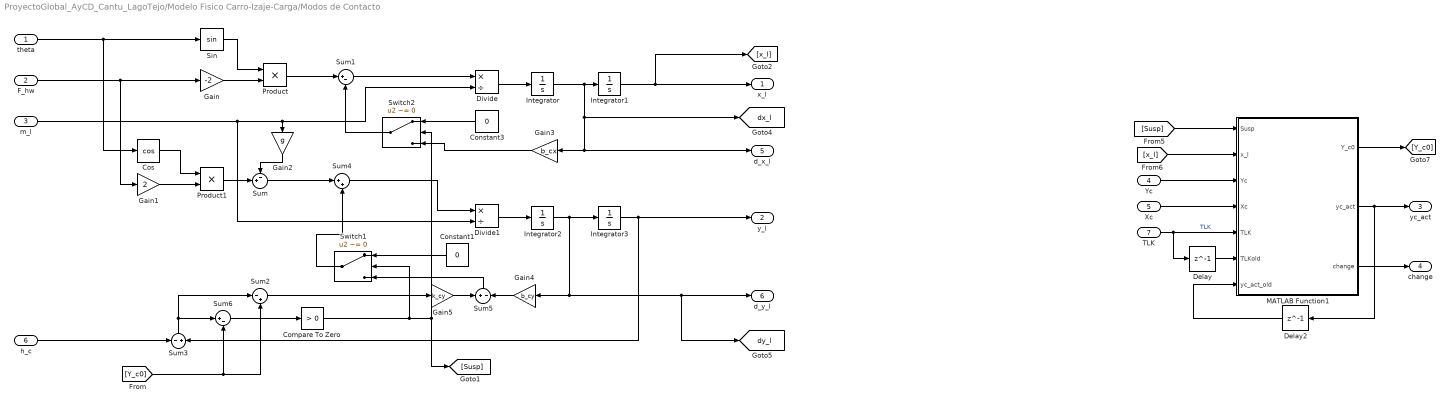
== system ProyectoGlobal_AyCD_Cantu_LagoTejo/Modelo Fisico Carro-Izaje-Carga/Modos de Contacto ==
  theta : Inport
  F_hw : Inport  Port=2
  m_l : Inport  Port=3
  Yc : Inport  Port=4
  Xc : Inport  Port=5
  h_c : Inport  Port=6
  TLK : Inport  Port=7
  Compare To Zero : simulink/Logic and Bit Operations/Compare To Zero  relop=>  OutDataTypeStr=boolean
  Constant1 : Constant  Value=0
  Constant3 : Constant  Value=0
  Cos : Trigonometry  Operator=cos
  Delay : Delay  DelayLength=1
  Delay2 : Delay  DelayLength=1
  Divide : Product  Inputs=*/
  Divide1 : Product  Inputs=*/
  Gain : Gain  Gain=-2
  Gain1 : Gain  Gain=2
  Gain2 : Gain  Gain=g
  Gain3 : Gain  Gain=b_cx
  Gain4 : Gain  Gain=b_cy
  Gain5 : Gain  Gain=k_cy
  Integrator : Integrator
  Integrator1 : Integrator  InitialCondition=CI_t
  Integrator2 : Integrator
  Integrator3 : Integrator  InitialCondition=CI_h
  MATLAB Function1 : MATLAB Function  TreatAsAtomicUnit=on
  Product : Product
  Product1 : Product
  Sin : Trigonometry
  Sum : Sum  Inputs=-+|
  Sum1 : Sum  Inputs=|+-
  Sum2 : Sum  Inputs=|-+
  Sum3 : Sum  Inputs=-|+
  Sum4 : Sum  Inputs=|++
  Sum5 : Sum  Inputs=+|-
  Sum6 : Sum  Inputs=|+-
  Switch1 : Switch  Criteria=u2 ~= 0
  Switch2 : Switch  Criteria=u2 ~= 0
  x_l : Outport
  y_l : Outport  Port=2
  yc_act : Outport  Port=3
  change : Outport  Port=4
  d_x_l : Outport  Port=5
  d_y_l : Outport  Port=6
  tag scope: dx_l=global, dy_l=global
  wires:
  Gain/1 -> Product/2
  Sin/1 -> Product/1
  Cos/1 -> Product1/1
  Gain1/1 -> Product1/2
  Divide/1 -> Integrator/1
  Integrator/1 -> Integrator1/1, d_x_l/1, Gain3/1, [dx_l]
  Divide1/1 -> Integrator2/1
  Integrator2/1 -> [dy_l], d_y_l/1, Gain4/1, Integrator3/1
  Integrator3/1 -> Sum3/2, y_l/1
  Product/1 -> Sum1/1
  Sum1/1 -> Divide/1
  Switch2/1 -> Sum1/2
  Constant3/1 -> Switch2/1
  Gain3/1 -> Switch2/3
  Sum5/1 -> Switch1/3
  Gain5/1 -> Sum5/1
  Gain4/1 -> Sum5/2
  Constant1/1 -> Switch1/1
  h_c/1 -> Sum3/1
  Sum3/1 -> Sum6/1, Sum2/1
  Sum/1 -> Sum4/1
  Sum4/1 -> Divide1/1
  Switch1/1 -> Sum4/2
  Product1/1 -> Sum/2
  Gain2/1 -> Sum/1
  Integrator1/1 -> [x_l], x_l/1
  Sum2/1 -> Gain5/1
  Sum6/1 -> Compare To Zero/1
  F_hw/1 -> Gain/1, Gain1/1
  Compare To Zero/1 -> [Susp], Switch2/2, Switch1/2
  TLK/1 -> Delay/1, MATLAB Function1/5(TLK)  "TLK"
  Yc/1 -> MATLAB Function1/3(Yc)
  Xc/1 -> MATLAB Function1/4(Xc)
  m_l/1 -> Divide/2, Gain2/1, Divide1/2
  MATLAB Function1/2(yc_act) -> yc_act/1, Delay2/1
  MATLAB Function1/3(change) -> change/1
  Delay2/1 -> MATLAB Function1/7(yc_act_old)
  [x_l] -> MATLAB Function1/2(x_l)
  [Susp] -> MATLAB Function1/1(Susp)
  MATLAB Function1/1(Y_c0) -> [Y_c0]
  Delay/1 -> MATLAB Function1/6(TLKold)
  theta/1 -> Sin/1, Cos/1
  [Y_c0] -> Sum2/2, Sum6/2

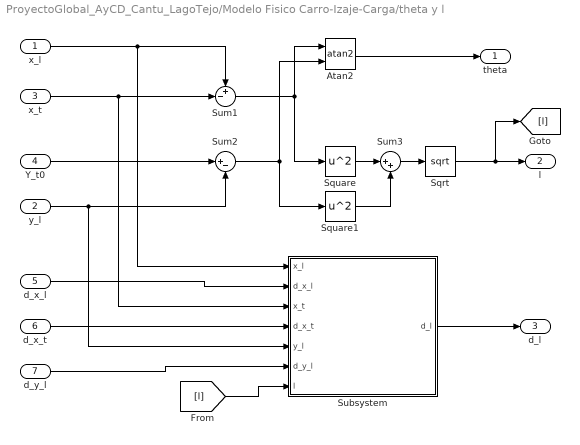
== system ProyectoGlobal_AyCD_Cantu_LagoTejo/Modelo Fisico Carro-Izaje-Carga/theta y l ==
  x_l : Inport
  y_l : Inport  Port=2
  x_t : Inport  Port=3
  Y_t0 : Inport  Port=4
  d_x_l : Inport  Port=5
  d_x_t : Inport  Port=6
  d_y_l : Inport  Port=7
  Atan2 : Trigonometry  Operator=atan2
  Sqrt : Sqrt  SaturateOnIntegerOverflow=on
  Square : Math  Operator=square  SaturateOnIntegerOverflow=on
  Square1 : Math  Operator=square  SaturateOnIntegerOverflow=on
  Subsystem : Subsystem
  Sum1 : Sum  Inputs=+-|
  Sum2 : Sum  Inputs=|+-
  Sum3 : Sum  Inputs=|++
  theta : Outport
  l : Outport  Port=2
  d_l : Outport  Port=3
  wires:
  x_l/1 -> Subsystem/1(x_l), Sum1/1
  x_t/1 -> Subsystem/3(x_t), Sum1/2
  Y_t0/1 -> Sum2/1
  y_l/1 -> Subsystem/5(y_l), Sum2/2
  Sum1/1 -> Square/1, Atan2/1
  Sum2/1 -> Square1/1, Atan2/2
  Sum3/1 -> Sqrt/1
  Sqrt/1 -> [l], l/1
  Square/1 -> Sum3/1
  Square1/1 -> Sum3/2
  Atan2/1 -> theta/1
  [l] -> Subsystem/7(l)
  d_x_l/1 -> Subsystem/2(d_x_l)
  d_x_t/1 -> Subsystem/4(d_x_t)
  d_y_l/1 -> Subsystem/6(d_y_l)
  Subsystem/1(d_l) -> d_l/1

== system ProyectoGlobal_AyCD_Cantu_LagoTejo/Nivel 2/Control PD Balanceo ==
  Kp_bal : Inport
  Kd_bal : Inport  Port=2
  theta : Inport  Port=3
  Constant2 : Constant  Value=0
  Delay One Step : Delay  DelayLength=1  SampleTime=1e-3
  Gain1 : Gain  Gain=1/d_t
  Product : Product
  Product1 : Product
  Sum1 : Sum  Inputs=|+-
  Sum2 : Sum  Inputs=|+-
  Sum3 : Sum  Inputs=++|
  d_x_t* : Outport
  wires:
  Product1/1 -> Sum3/2
  Gain1/1 -> Product/2
  Product/1 -> Sum3/1
  Sum2/1 -> Gain1/1
  Constant2/1 -> Sum1/1
  Sum1/1 -> Product1/2, Sum2/1, Delay One Step/1
  Delay One Step/1 -> Sum2/2
  theta/1 -> Sum1/2
  Sum3/1 -> d_x_t*/1
  Kp_bal/1 -> Product1/1
  Kd_bal/1 -> Product/1

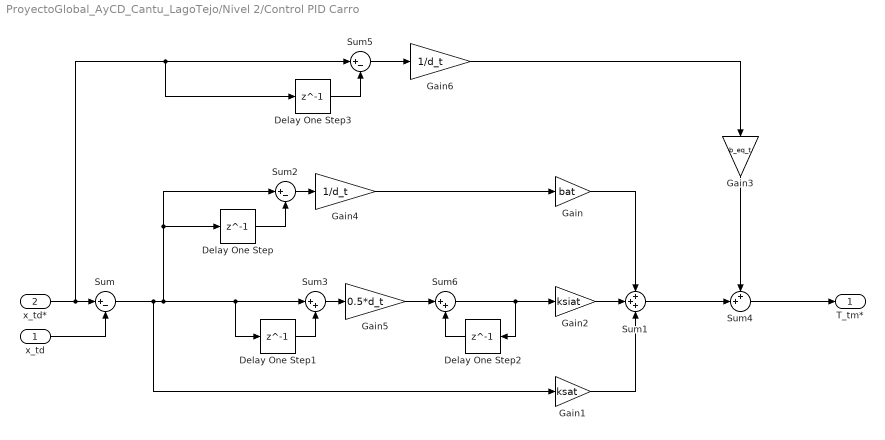
== system ProyectoGlobal_AyCD_Cantu_LagoTejo/Nivel 2/Control PID Carro ==
  x_td : Inport
  x_td* : Inport  Port=2
  Delay One Step{,1..3} (4 alike) : Delay  DelayLength=1  SampleTime=1e-3
  Gain : Gain  Gain=bat
  Gain1 : Gain  Gain=ksat
  Gain2 : Gain  Gain=ksiat
  Gain3 : Gain  Gain=b_eq_t
  Gain4 : Gain  Gain=1/d_t
  Gain5 : Gain  Gain=0.5*d_t
  Gain6 : Gain  Gain=1/d_t
  Sum : Sum  Inputs=|+-
  Sum1 : Sum  Inputs=+++
  Sum2 : Sum  Inputs=|+-
  Sum3 : Sum  Inputs=|++
  Sum4 : Sum  Inputs=++|
  Sum5 : Sum  Inputs=|+-
  Sum6 : Sum  Inputs=|++
  T_tm* : Outport
  wires:
  Gain5/1 -> Sum6/1
  Sum1/1 -> Sum4/2
  Gain1/1 -> Sum1/3
  x_td/1 -> Sum/2
  Delay One Step3/1 -> Sum5/2
  Gain3/1 -> Sum4/1
  Sum5/1 -> Gain6/1
  Gain6/1 -> Gain3/1
  x_td*/1 -> Delay One Step3/1, Sum5/1, Sum/1
  Sum/1 -> Delay One Step/1, Sum2/1, Delay One Step1/1, Sum3/1, Gain1/1
  Delay One Step1/1 -> Sum3/2
  Sum2/1 -> Gain4/1
  Delay One Step/1 -> Sum2/2
  Sum4/1 -> T_tm*/1
  Gain4/1 -> Gain/1
  Gain/1 -> Sum1/1
  Gain2/1 -> Sum1/2
  Sum3/1 -> Gain5/1
  Delay One Step2/1 -> Sum6/2
  Sum6/1 -> Delay One Step2/1, Gain2/1

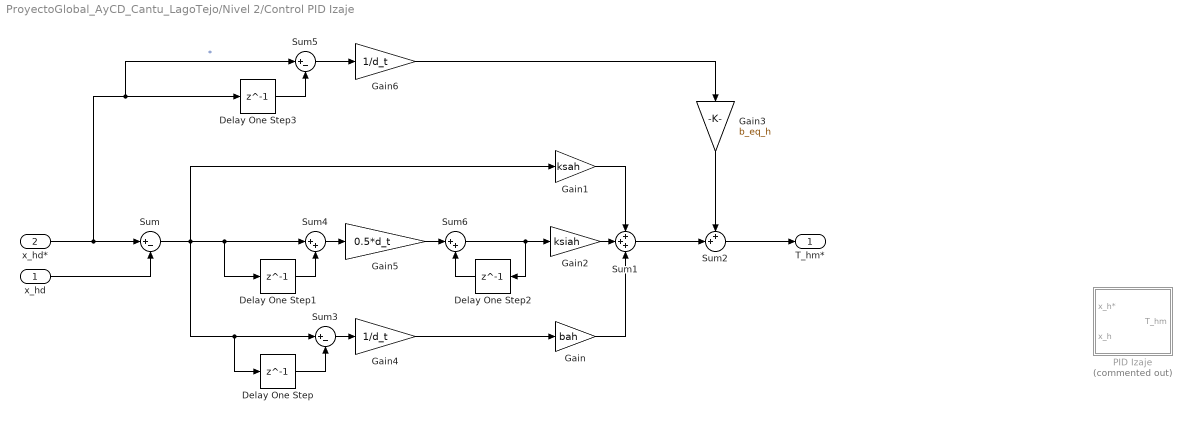
== system ProyectoGlobal_AyCD_Cantu_LagoTejo/Nivel 2/Control PID Izaje ==
  x_hd : Inport
  x_hd* : Inport  Port=2
  Delay One Step{,1..3} (4 alike) : Delay  DelayLength=1  SampleTime=1e-3
  Gain : Gain  Gain=bah
  Gain1 : Gain  Gain=ksah
  Gain2 : Gain  Gain=ksiah
  Gain3 : Gain  Gain=b_eq_h
  Gain4 : Gain  Gain=1/d_t
  Gain5 : Gain  Gain=0.5*d_t
  Gain6 : Gain  Gain=1/d_t
  PID Izaje : Subsystem  Commented=on
  Sum : Sum  Inputs=|+-
  Sum1 : Sum  Inputs=+++
  Sum2 : Sum  Inputs=++|
  Sum3 : Sum  Inputs=|+-
  Sum4 : Sum  Inputs=|++
  Sum5 : Sum  Inputs=|+-
  Sum6 : Sum  Inputs=|++
  T_hm* : Outport
  wires:
  Gain4/1 -> Gain/1
  Delay One Step3/1 -> Sum5/2
  Gain1/1 -> Sum1/1
  Gain6/1 -> Gain3/1
  Gain3/1 -> Sum2/1
  Sum6/1 -> Gain2/1, Delay One Step2/1
  Sum1/1 -> Sum2/2
  x_hd*/1 -> Sum/1, Sum5/1, Delay One Step3/1  "*"
  Gain5/1 -> Sum6/1
  Delay One Step1/1 -> Sum4/2
  Delay One Step/1 -> Sum3/2
  x_hd/1 -> Sum/2
  Delay One Step2/1 -> Sum6/2
  Sum2/1 -> T_hm*/1
  Gain2/1 -> Sum1/2
  Sum3/1 -> Gain4/1
  Gain/1 -> Sum1/3
  Sum/1 -> Delay One Step1/1, Sum4/1, Delay One Step/1, Sum3/1, Gain1/1
  Sum4/1 -> Gain5/1
  Sum5/1 -> Gain6/1

== system ProyectoGlobal_AyCD_Cantu_LagoTejo/Nivel 2/Mod Torque Carro ==
  T_tm* : Inport
  Filtro PB 1° Orden : StateSpace  A=-1/tau_tm  C=1/tau_tm  D=0  InitialCondition=0
  T_tmMax : Saturate  UpperLimit=T_tmMax  LowerLimit=-T_tmMax
  T_tm : Outport
  wires:
  T_tm*/1 -> Filtro PB 1° Orden/1
  Filtro PB 1° Orden/1 -> T_tmMax/1
  T_tmMax/1 -> T_tm/1

== system ProyectoGlobal_AyCD_Cantu_LagoTejo/Nivel 2/Mod Torque Carro1 ==
  T_tm* : Inport
  Gain : Gain  Gain=1/tau_tm
  Integrator : Integrator  InitialConditionSource=external
  Sum : Sum  Inputs=|+-
  T_tmMax : Saturate  UpperLimit=T_tmMax  LowerLimit=-T_tmMax
  T_tm : Outport
  wires:
  T_tm*/1 -> T_tmMax/1
  Gain/1 -> Integrator/1
  Integrator/1 -> T_tm/1, Sum/2
  Sum/1 -> Gain/1
  T_tmMax/1 -> Integrator/2, Sum/1

== system ProyectoGlobal_AyCD_Cantu_LagoTejo/Nivel 2/Mod Torque Izaje ==
  T_hm* : Inport
  Filtro PB 1° Orden : StateSpace  A=-1/tau_hm  C=1/tau_hm  D=0  InitialCondition=0  ParameterTunability=Unconstrained
  T_hmMax : Saturate  UpperLimit=T_hmMax  LowerLimit=-T_hmMax
  T_hm : Outport
  wires:
  T_hm*/1 -> Filtro PB 1° Orden/1
  Filtro PB 1° Orden/1 -> T_hmMax/1
  T_hmMax/1 -> T_hm/1

== system ProyectoGlobal_AyCD_Cantu_LagoTejo/Nivel 2/Mod Torque Izaje1 ==
  T_hm* : Inport
  Gain : Gain  Gain=1/tau_hm
  Integrator : Integrator  InitialConditionSource=external
  Sum : Sum  Inputs=|+-
  T_hmMax : Saturate  UpperLimit=T_hmMax  LowerLimit=-T_hmMax
  T_hm : Outport
  wires:
  T_hm*/1 -> T_hmMax/1
  Gain/1 -> Integrator/1
  Integrator/1 -> T_hm/1, Sum/2
  Sum/1 -> Gain/1
  T_hmMax/1 -> Integrator/2, Sum/1

== system ProyectoGlobal_AyCD_Cantu_LagoTejo/Nivel 2/Subsystem2 ==
  d_x_hd : Inport
  AND : Logic  Operator=NAND  Inputs=3  IconShape=distinctive  AllPortsSameDT=off  OutDataTypeStr=boolean
  Abs1 : Abs
  Abs2 : Abs
  Abs3 : Abs
  Compare To Constant1 : simulink/Logic and Bit Operations/Compare To Constant  relop=<  const=1e-2  OutDataTypeStr=boolean
  Compare To Constant2 : simulink/Logic and Bit Operations/Compare To Constant  relop=<  const=1e-2  OutDataTypeStr=boolean
  Compare To Constant3 : simulink/Logic and Bit Operations/Compare To Constant  relop=<  const=1e-2  OutDataTypeStr=boolean
  Memory : Memory
  Memory1 : Memory
  vel_h_on : Outport
  wires:
  Abs1/1 -> Compare To Constant1/1
  d_x_hd/1 -> Abs1/1, Memory/1
  Abs2/1 -> Compare To Constant2/1
  Memory/1 -> Abs2/1, Memory1/1
  Abs3/1 -> Compare To Constant3/1
  Memory1/1 -> Abs3/1
  Compare To Constant1/1 -> AND/1
  Compare To Constant2/1 -> AND/2
  Compare To Constant3/1 -> AND/3
  AND/1 -> vel_h_on/1

== system ProyectoGlobal_AyCD_Cantu_LagoTejo/Nivel 2/Subsystem3 ==
  d_x_td : Inport
  AND : Logic  Operator=NAND  Inputs=3  IconShape=distinctive  AllPortsSameDT=off  OutDataTypeStr=boolean
  Abs1 : Abs
  Abs2 : Abs
  Abs3 : Abs
  Compare To Constant1 : simulink/Logic and Bit Operations/Compare To Constant  relop=<  const=1e-2  OutDataTypeStr=boolean
  Compare To Constant2 : simulink/Logic and Bit Operations/Compare To Constant  relop=<  const=1e-2  OutDataTypeStr=boolean
  Compare To Constant3 : simulink/Logic and Bit Operations/Compare To Constant  relop=<  const=1e-2  OutDataTypeStr=boolean
  Memory : Memory
  Memory1 : Memory
  vel_t_on : Outport
  wires:
  Abs1/1 -> Compare To Constant1/1
  d_x_td/1 -> Abs1/1, Memory/1
  Abs2/1 -> Compare To Constant2/1
  Memory/1 -> Abs2/1, Memory1/1
  Abs3/1 -> Compare To Constant3/1
  Memory1/1 -> Abs3/1
  Compare To Constant1/1 -> AND/1
  Compare To Constant2/1 -> AND/2
  Compare To Constant3/1 -> AND/3
  AND/1 -> vel_t_on/1

== system ProyectoGlobal_AyCD_Cantu_LagoTejo/Modelo Fisico Carro-Izaje-Carga/Carro/Carro Eje Rápido-Lento ==
  F_tw : Inport
  T_tb : Inport  Port=2
  T_tm : Inport  Port=3
  1/M_eq_t : Gain  Gain=1/M_eq_td
  Gain3 : Gain  Gain=i_t/r_td
  Integrator2 : Integrator
  Integrator3 : Integrator  InitialCondition=CI_t
  Sum : Sum  Inputs=|++
  Sum1 : Sum  Inputs=-+-
  b_eq_t : Gain  Gain=b_eq_td
  x_td : Outport
  d_x_td : Outport  Port=2
  wires:
  Integrator2/1 -> d_x_td/1, b_eq_t/1, Integrator3/1
  Integrator3/1 -> x_td/1
  1/M_eq_t/1 -> Integrator2/1
  Sum1/1 -> 1/M_eq_t/1
  b_eq_t/1 -> Sum1/3
  F_tw/1 -> Sum1/1
  T_tm/1 -> Sum/1
  T_tb/1 -> Sum/2
  Sum/1 -> Gain3/1
  Gain3/1 -> Sum1/2
